simulink model "untitled"  (R2015a)
settings: Solver=ode45  StartTime=0.0  StopTime=1000.0  RelTol=1e-3
libraries: commchan3 x2, commdigbbndpm3 x2, commsink2 x2, commrandsrc2 x1
settings Model: Creator=francisco  LastModifiedBy=francisco

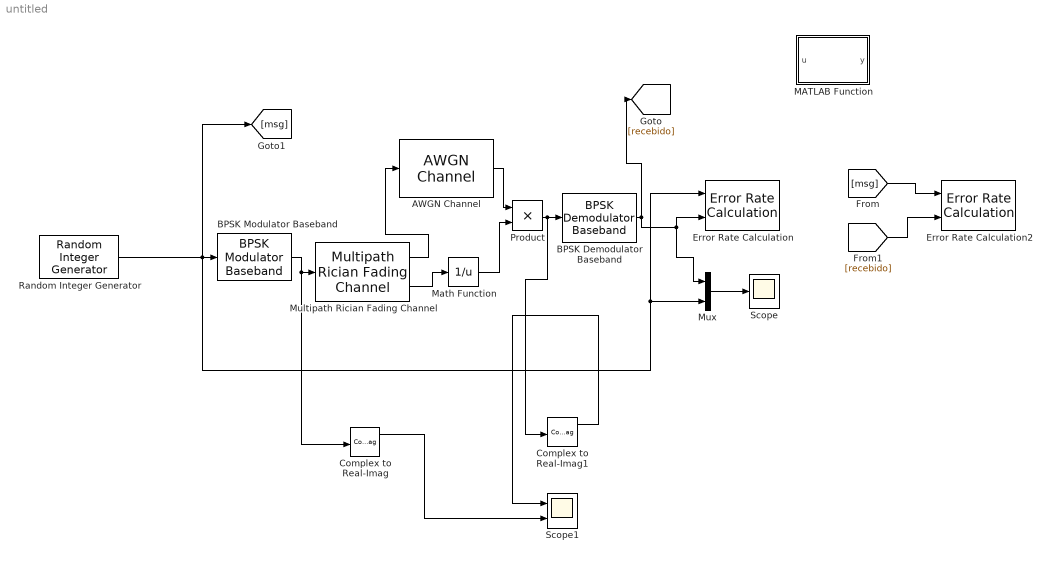
== system untitled ==
  AWGN Channel : commchan3/AWGN Channel  InputProcessing=Columns as channels (frame based)  seed=67  noiseMode="Signal to noise ratio  (Eb/No)"  EbNodB=40  EsNodB=10  SNRdB=10  bitsPerSym=1  Ps=1  Tsym=1  variance=1
  BPSK Demodulator Baseband : commdigbbndpm3/BPSK Demodulator Baseband  Ph=0  DecType=Hard decision  VarSource=Dialog  Variance=1  outDtype=Inherit via internal rule  derotateFactorWordLen=16
  BPSK Modulator Baseband : commdigbbndpm3/BPSK Modulator Baseband  Ph=0  outDtype=double  outWordLen=16  outUDDataType=sfix(16)  outFracLenMode=Best precision  outFracLen=15
  Complex to Real-Imag : ComplexToRealImag
  Complex to Real-Imag1 : ComplexToRealImag
  Error Rate Calculation : commsink2/Error Rate Calculation  N=0  st_delay=0  cp_mode=Entire frame  subframe=[]  PMode=Workspace  WsName=ErrorVec  RsMode2=off  stop=off  numErr=100  maxBits=1e6
  Error Rate Calculation2 : commsink2/Error Rate Calculation  N=0  st_delay=0  cp_mode=Entire frame  subframe=[]  PMode=Port  WsName=ErrorVec  RsMode2=off  stop=off  numErr=100  maxBits=1e6
  MATLAB Function : MATLAB Function  TreatAsAtomicUnit=on
  Math Function : Math  Operator=reciprocal  SaturateOnIntegerOverflow=on
  Multipath Rician Fading Channel : commchan3/Multipath Rician Fading Channel  K=100  fdLOS=0.01  thetaLOS=0  maxDopplerShift=0.1  spectrumType=Jakes  sigmaGaussian=1/sqrt(2)  coeffRounded=[1 -1.72 0.785]  freqMinMaxRJakes=[0 1]  freqMinMaxAJakes=[0 1]  sigmaGaussian1=1/sqrt(2)  sigmaGaussian2=1/sqrt(2)  centerFreqGaussian1=0  centerFreqGaussian2=0  gainGaussian1=0.5  gainGaussian2=0.5  coeffBell=9  dopplerSpectrum=doppler.jakes  pathDelays=0  avgPathGaindB=0  normalizePathGains=on  seed=73  enableProbe=0  openVisAtStart=off  outPathGains=on  outDelay=off
  Mux : Mux  Inputs=2
  Product : Product
  Random Integer Generator : commrandsrc2/Random Integer Generator  mul=2  seed=37  Ts=0.01  frameBased=off  sampPerFrame=1  orient=off  outDataType=double
  Scope : Scope
      settings: Decimation=100
  Scope1 : Scope  NumInputPorts=2
      settings: TimeRange=1000  YMin=-5~-5  YMax=5~5  Decimation=100
  wires:
  Random Integer Generator/1 -> [msg], BPSK Modulator Baseband/1, Error Rate Calculation/1, Mux/2
  BPSK Demodulator Baseband/1 -> Mux/1, Error Rate Calculation/2, [recebido]
  Mux/1 -> Scope/1
  BPSK Modulator Baseband/1 -> Complex to Real-Imag/1, Multipath Rician Fading Channel/1
  Multipath Rician Fading Channel/1 -> AWGN Channel/1
  Complex to Real-Imag1/1 -> Scope1/1
  Complex to Real-Imag/1 -> Scope1/2
  [msg] -> Error Rate Calculation2/1
  [recebido] -> Error Rate Calculation2/2
  Multipath Rician Fading Channel/2 -> Math Function/1
  AWGN Channel/1 -> Product/1
  Math Function/1 -> Product/2
  Product/1 -> Complex to Real-Imag1/1, BPSK Demodulator Baseband/1

== matlab function untitled/MATLAB Function ==
  data: u input; y output
function y = fcn(u)
%#codegen

y = u;
